simulink library "fuelCellLibrary"  (R2020b)
settings: Solver=VariableStepAuto  StartTime=0.0  StopTime=10.0  RelTol=1e-3
undefined symbols (not defined in the file): fuelCell
settings Model: Creator=ericb  LastModifiedBy=ericb

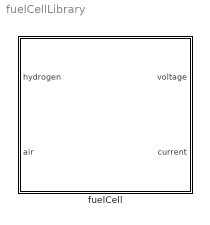
== system fuelCellLibrary ==
  fuelCell : Subsystem  Variant=on

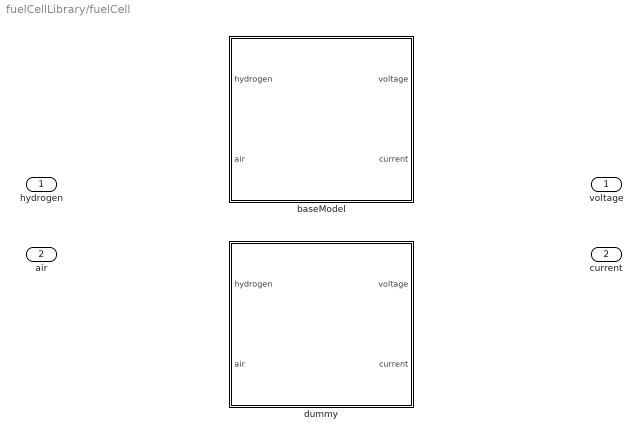
== system fuelCellLibrary/fuelCell ==
  hydrogen : Inport
  air : Inport  Port=2
  baseModel : Subsystem  VariantControl=strcmp(fuelCell.blockChoice,'baseModel')
  dummy : Subsystem  VariantControl=strcmp(fuelCell.blockChoice,'dummy')
  voltage : Outport
  current : Outport  Port=2

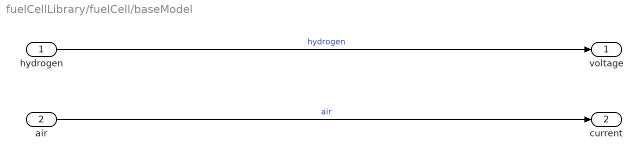
== system fuelCellLibrary/fuelCell/baseModel ==
  hydrogen : Inport
  air : Inport  Port=2
  voltage : Outport
  current : Outport  Port=2
  wires:
  hydrogen/1 -> voltage/1  "hydrogen"
  air/1 -> current/1  "air"

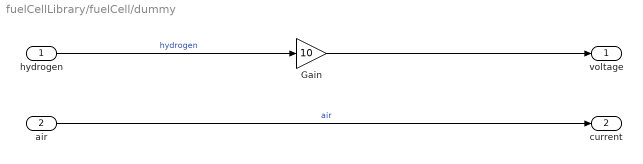
== system fuelCellLibrary/fuelCell/dummy ==
  hydrogen : Inport
  air : Inport  Port=2
  Gain : Gain  Gain=10
  voltage : Outport
  current : Outport  Port=2
  wires:
  hydrogen/1 -> Gain/1  "hydrogen"
  Gain/1 -> voltage/1
  air/1 -> current/1  "air"
